simulink model "boat_control"  (R2018b)
settings: Solver=VariableStepAuto  StartTime=0.0  StopTime=150  RelTol=1e-3
libraries: simulink x5
settings Model: PacingRate=0.890000  Creator=davidm  LastModifiedBy=davidm

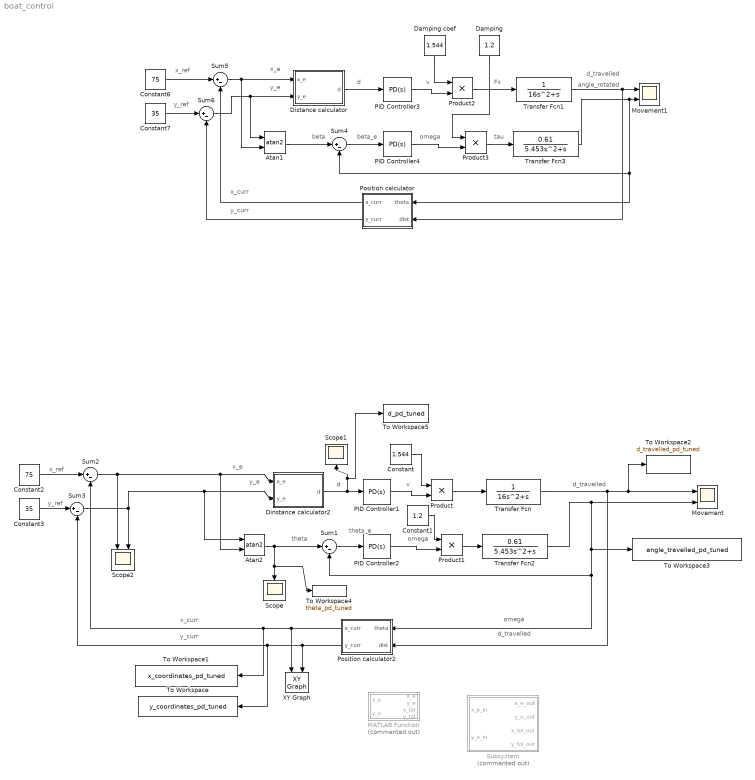
== system boat_control ==
  note: angle_rotated
  note: Fx
  note: tau
  note: y_curr
  note: x_curr
  note: omega
  note: theta
  note: d_travelled
  note: v
  note: d
  note: y_e
  note: x_e
  note: y_ref
  note: x_ref
  note: theta_e
  note: omega
  note: d_travelled
  note: y_e
  note: x_e
  note: d
  note: y_ref
  note: v
  note: d_travelled
  note: beta_e
  note: x_ref
  note: beta
  note: omega
  note: x_curr
  note: y_curr
  Atan1 : Trigonometry  Operator=atan2
  Atan2 : Trigonometry  Operator=atan2
  Constant : Constant  Value=1.544
  Constant1 : Constant  Value=1.2
  Constant2 : Constant  Value=75
  Constant3 : Constant  Value=35
  Constant6 : Constant  Value=75
  Constant7 : Constant  Value=35
  Damping : Constant  Value=1.2
  Damping coef : Constant  Value=1.544
  Dinstance calculator2 : MATLAB Function  TreatAsAtomicUnit=on
  Distance calculator : MATLAB Function  TreatAsAtomicUnit=on
  MATLAB Function : MATLAB Function  Commented=on  TreatAsAtomicUnit=on
  Movement : Scope  NumInputPorts=2
  Movement1 : Scope  NumInputPorts=2
  PID Controller1 : simulink/Continuous/PID Controller  Controller=PD  Form=Parallel  TimeDomain=Continuous-time  SampleTime=-1  IntegratorMethod=Forward Euler  FilterMethod=Forward Euler  ControllerParametersSource=internal  P=0.115276413128131  I=0.00135505762416607  D=0.95237367994795  UseFilter=on  N=1.3850682547936  TunerSelectOption=Transfer Function Based (PID Tuner App)  InitialConditionSource=internal  InitialConditionForIntegrator=0  InitialConditionForFilter=0  DifferentiatorICPrevScaledInput=0  ExternalReset=none  TrackingMode=off  Kt=1  LimitOutput=off  UpperSaturationLimit=inf  LowerSaturationLimit=-inf  LinearizeAsGain=on  AntiWindupMode=clamping  Kb=1  POutMin=[]  POutMax=[]  IOutMin=[]  IOutMax=[]  DOutMin=[]  DOutMax=[]  NOutMin=[]  NOutMax=[]  SumOutMin=[]  SumOutMax=[]  SaturationOutMin=[]  SaturationOutMax=[]  PParamMin=[]  PParamMax=[]  IParamMin=[]  IParamMax=[]  DParamMin=[]  DParamMax=[]  NParamMin=[]  NParamMax=[]  KbParamMin=[]  KbParamMax=[]  KtParamMin=[]  KtParamMax=[]  KbOutMin=[]  KbOutMax=[]  KtOutMin=[]  KtOutMax=[]  IntegratorOutMin=[]  IntegratorOutMax=[]  FilterOutMin=[]  FilterOutMax=[]  SumI1OutMin=[]  SumI1OutMax=[]  SumI2OutMin=[]  SumI2OutMax=[]  SumI3OutMin=[]  SumI3OutMax=[]  SumI4OutMin=[]  SumI4OutMax=[]  SumDOutMin=[]  SumDOutMax=[]  DifferentiatorOutMin=[]  DifferentiatorOutMax=[]  FilterDiffOutCoefMin=[]  FilterDiffOutCoefMax=[]  ReciprocalOutMin=[]  ReciprocalOutMax=[]  SumDenOutMin=[]  SumDenOutMax=[]  SumNumOutMin=[]  SumNumOutMax=[]  DivideOutMin=[]  DivideOutMax=[]  IntegratorContinuousStateAttributes=''  IntegratorStateMustResolveToSignalObject=off  IntegratorRTWStateStorageClass=Auto  FilterContinuousStateAttributes=''  FilterStateMustResolveToSignalObject=off  FilterRTWStateStorageClass=Auto  ParallelPVariant=InternalParameters  IdealPVariant=Disabled  IVariant=Disabled  DVariant=InternalParameters  IntegratorVariant=Disabled  SatVariant=Disabled  AWVariant=Disabled  PCopyVariant=Disabled  TRVariant=Disabled  FdbkBlocksVariant=Forward  IdealPFdbkVariant=Disabled  SatFdbkVariant=Disabled  DerivativeFilterVariant=ContFilter  NVariant=InternalParameters  NCopyVariant=Disabled  FilterICVariant=InternalICsFilter  IntegratorICVariant=Disabled  ExternalResetVariant=Disabled  TRSumVariant=Passthrough  SumFdbkVariant=Disabled  SumVariant=Sum_PD
  PID Controller2 : simulink/Continuous/PID Controller  Controller=PD  Form=Parallel  TimeDomain=Continuous-time  SampleTime=-1  IntegratorMethod=Forward Euler  FilterMethod=Forward Euler  ControllerParametersSource=internal  P=0.646512806885205  I=0.022298668264277  D=1.82036961249766  UseFilter=on  N=4.06401835259447  TunerSelectOption=Transfer Function Based (PID Tuner App)  InitialConditionSource=internal  InitialConditionForIntegrator=0  InitialConditionForFilter=0  DifferentiatorICPrevScaledInput=0  ExternalReset=none  TrackingMode=off  Kt=1  LimitOutput=off  UpperSaturationLimit=inf  LowerSaturationLimit=-inf  LinearizeAsGain=off  AntiWindupMode=clamping  Kb=1  POutMin=[]  POutMax=[]  IOutMin=[]  IOutMax=[]  DOutMin=[]  DOutMax=[]  NOutMin=[]  NOutMax=[]  SumOutMin=[]  SumOutMax=[]  SaturationOutMin=[]  SaturationOutMax=[]  PParamMin=[]  PParamMax=[]  IParamMin=[]  IParamMax=[]  DParamMin=[]  DParamMax=[]  NParamMin=[]  NParamMax=[]  KbParamMin=[]  KbParamMax=[]  KtParamMin=[]  KtParamMax=[]  KbOutMin=[]  KbOutMax=[]  KtOutMin=[]  KtOutMax=[]  IntegratorOutMin=[]  IntegratorOutMax=[]  FilterOutMin=[]  FilterOutMax=[]  SumI1OutMin=[]  SumI1OutMax=[]  SumI2OutMin=[]  SumI2OutMax=[]  SumI3OutMin=[]  SumI3OutMax=[]  SumI4OutMin=[]  SumI4OutMax=[]  SumDOutMin=[]  SumDOutMax=[]  DifferentiatorOutMin=[]  DifferentiatorOutMax=[]  FilterDiffOutCoefMin=[]  FilterDiffOutCoefMax=[]  ReciprocalOutMin=[]  ReciprocalOutMax=[]  SumDenOutMin=[]  SumDenOutMax=[]  SumNumOutMin=[]  SumNumOutMax=[]  DivideOutMin=[]  DivideOutMax=[]  IntegratorContinuousStateAttributes=''  IntegratorStateMustResolveToSignalObject=off  IntegratorRTWStateStorageClass=Auto  FilterContinuousStateAttributes=''  FilterStateMustResolveToSignalObject=off  FilterRTWStateStorageClass=Auto  ParallelPVariant=InternalParameters  IdealPVariant=Disabled  IVariant=Disabled  DVariant=InternalParameters  IntegratorVariant=Disabled  SatVariant=Disabled  AWVariant=Disabled  PCopyVariant=Disabled  TRVariant=Disabled  FdbkBlocksVariant=Forward  IdealPFdbkVariant=Disabled  SatFdbkVariant=Disabled  DerivativeFilterVariant=ContFilter  NVariant=InternalParameters  NCopyVariant=Disabled  FilterICVariant=InternalICsFilter  IntegratorICVariant=Disabled  ExternalResetVariant=Disabled  TRSumVariant=Passthrough  SumFdbkVariant=Disabled  SumVariant=Sum_PD
  PID Controller3 : simulink/Continuous/PID Controller  Controller=PD  Form=Parallel  TimeDomain=Continuous-time  SampleTime=-1  IntegratorMethod=Forward Euler  FilterMethod=Forward Euler  ControllerParametersSource=internal  P=0.0932700762153962  I=0.00135505762416607  D=1.11983436282053  UseFilter=on  N=0.405940642828316  TunerSelectOption=Transfer Function Based (PID Tuner App)  InitialConditionSource=internal  InitialConditionForIntegrator=0  InitialConditionForFilter=0  DifferentiatorICPrevScaledInput=0  ExternalReset=none  TrackingMode=off  Kt=1  LimitOutput=off  UpperSaturationLimit=inf  LowerSaturationLimit=-inf  LinearizeAsGain=on  AntiWindupMode=clamping  Kb=1  POutMin=[]  POutMax=[]  IOutMin=[]  IOutMax=[]  DOutMin=[]  DOutMax=[]  NOutMin=[]  NOutMax=[]  SumOutMin=[]  SumOutMax=[]  SaturationOutMin=[]  SaturationOutMax=[]  PParamMin=[]  PParamMax=[]  IParamMin=[]  IParamMax=[]  DParamMin=[]  DParamMax=[]  NParamMin=[]  NParamMax=[]  KbParamMin=[]  KbParamMax=[]  KtParamMin=[]  KtParamMax=[]  KbOutMin=[]  KbOutMax=[]  KtOutMin=[]  KtOutMax=[]  IntegratorOutMin=[]  IntegratorOutMax=[]  FilterOutMin=[]  FilterOutMax=[]  SumI1OutMin=[]  SumI1OutMax=[]  SumI2OutMin=[]  SumI2OutMax=[]  SumI3OutMin=[]  SumI3OutMax=[]  SumI4OutMin=[]  SumI4OutMax=[]  SumDOutMin=[]  SumDOutMax=[]  DifferentiatorOutMin=[]  DifferentiatorOutMax=[]  FilterDiffOutCoefMin=[]  FilterDiffOutCoefMax=[]  ReciprocalOutMin=[]  ReciprocalOutMax=[]  SumDenOutMin=[]  SumDenOutMax=[]  SumNumOutMin=[]  SumNumOutMax=[]  DivideOutMin=[]  DivideOutMax=[]  IntegratorContinuousStateAttributes=''  IntegratorStateMustResolveToSignalObject=off  IntegratorRTWStateStorageClass=Auto  FilterContinuousStateAttributes=''  FilterStateMustResolveToSignalObject=off  FilterRTWStateStorageClass=Auto  ParallelPVariant=InternalParameters  IdealPVariant=Disabled  IVariant=Disabled  DVariant=InternalParameters  IntegratorVariant=Disabled  SatVariant=Disabled  AWVariant=Disabled  PCopyVariant=Disabled  TRVariant=Disabled  FdbkBlocksVariant=Forward  IdealPFdbkVariant=Disabled  SatFdbkVariant=Disabled  DerivativeFilterVariant=ContFilter  NVariant=InternalParameters  NCopyVariant=Disabled  FilterICVariant=InternalICsFilter  IntegratorICVariant=Disabled  ExternalResetVariant=Disabled  TRSumVariant=Passthrough  SumFdbkVariant=Disabled  SumVariant=Sum_PD
  PID Controller4 : simulink/Continuous/PID Controller  Controller=PD  Form=Parallel  TimeDomain=Continuous-time  SampleTime=-1  IntegratorMethod=Forward Euler  FilterMethod=Forward Euler  ControllerParametersSource=internal  P=0.52309312144704  I=0.022298668264277  D=2.1404544119915  UseFilter=on  N=1.19109669636036  TunerSelectOption=Transfer Function Based (PID Tuner App)  InitialConditionSource=internal  InitialConditionForIntegrator=0  InitialConditionForFilter=0  DifferentiatorICPrevScaledInput=0  ExternalReset=none  TrackingMode=off  Kt=1  LimitOutput=off  UpperSaturationLimit=inf  LowerSaturationLimit=-inf  LinearizeAsGain=off  AntiWindupMode=clamping  Kb=1  POutMin=[]  POutMax=[]  IOutMin=[]  IOutMax=[]  DOutMin=[]  DOutMax=[]  NOutMin=[]  NOutMax=[]  SumOutMin=[]  SumOutMax=[]  SaturationOutMin=[]  SaturationOutMax=[]  PParamMin=[]  PParamMax=[]  IParamMin=[]  IParamMax=[]  DParamMin=[]  DParamMax=[]  NParamMin=[]  NParamMax=[]  KbParamMin=[]  KbParamMax=[]  KtParamMin=[]  KtParamMax=[]  KbOutMin=[]  KbOutMax=[]  KtOutMin=[]  KtOutMax=[]  IntegratorOutMin=[]  IntegratorOutMax=[]  FilterOutMin=[]  FilterOutMax=[]  SumI1OutMin=[]  SumI1OutMax=[]  SumI2OutMin=[]  SumI2OutMax=[]  SumI3OutMin=[]  SumI3OutMax=[]  SumI4OutMin=[]  SumI4OutMax=[]  SumDOutMin=[]  SumDOutMax=[]  DifferentiatorOutMin=[]  DifferentiatorOutMax=[]  FilterDiffOutCoefMin=[]  FilterDiffOutCoefMax=[]  ReciprocalOutMin=[]  ReciprocalOutMax=[]  SumDenOutMin=[]  SumDenOutMax=[]  SumNumOutMin=[]  SumNumOutMax=[]  DivideOutMin=[]  DivideOutMax=[]  IntegratorContinuousStateAttributes=''  IntegratorStateMustResolveToSignalObject=off  IntegratorRTWStateStorageClass=Auto  FilterContinuousStateAttributes=''  FilterStateMustResolveToSignalObject=off  FilterRTWStateStorageClass=Auto  ParallelPVariant=InternalParameters  IdealPVariant=Disabled  IVariant=Disabled  DVariant=InternalParameters  IntegratorVariant=Disabled  SatVariant=Disabled  AWVariant=Disabled  PCopyVariant=Disabled  TRVariant=Disabled  FdbkBlocksVariant=Forward  IdealPFdbkVariant=Disabled  SatFdbkVariant=Disabled  DerivativeFilterVariant=ContFilter  NVariant=InternalParameters  NCopyVariant=Disabled  FilterICVariant=InternalICsFilter  IntegratorICVariant=Disabled  ExternalResetVariant=Disabled  TRSumVariant=Passthrough  SumFdbkVariant=Disabled  SumVariant=Sum_PD
  Position calculator : MATLAB Function  TreatAsAtomicUnit=on
  Position calculator2 : MATLAB Function  TreatAsAtomicUnit=on
  Product{,1..3} (4 alike) : Product
  Scope : Scope
  Scope1 : Scope
  Scope2 : Scope  NumInputPorts=2
  Subsystem : Subsystem  Commented=on
  Sum{1..6} (6 alike) : Sum  Inputs=|+-
  To Workspace : ToWorkspace  VariableName=y_coordinates_pd_tuned  SaveFormat=Timeseries  SampleTime=-1
  To Workspace1 : ToWorkspace  VariableName=x_coordinates_pd_tuned  SaveFormat=Timeseries  SampleTime=-1
  To Workspace2 : ToWorkspace  VariableName=d_travelled_pd_tuned  SaveFormat=Timeseries  SampleTime=-1
  To Workspace3 : ToWorkspace  VariableName=angle_travelled_pd_tuned  SaveFormat=Timeseries  SampleTime=-1
  To Workspace4 : ToWorkspace  VariableName=theta_pd_tuned  SaveFormat=Timeseries  SampleTime=-1
  To Workspace5 : ToWorkspace  VariableName=d_pd_tuned  SaveFormat=Timeseries  SampleTime=-1
  Transfer Fcn : TransferFcn  Denominator=[16 1 0]
  Transfer Fcn1 : TransferFcn  Denominator=[16 1 0]
  Transfer Fcn2 : TransferFcn  Numerator=[0.61]  Denominator=[5.453 1 0]
  Transfer Fcn3 : TransferFcn  Numerator=[0.61]  Denominator=[5.453 1 0]
  XY Graph : simulink/Sinks/XY Graph  xmin=0  xmax=5000  ymin=-150  ymax=150  st=-1
  wires:
  PID Controller1/1 -> Product/2
  Constant3/1 -> Sum3/1
  Constant2/1 -> Sum2/1
  Dinstance calculator2/1(d) -> PID Controller1/1, To Workspace5/1, Scope1/1
  Position calculator2/1(x_curr) -> XY Graph/1, To Workspace1/1, Sum2/2
  Position calculator2/2(y_curr) -> XY Graph/2, To Workspace/1, Sum3/2
  Transfer Fcn2/1 -> To Workspace3/1, Sum1/2, Position calculator2/1(theta), Movement/2
  Transfer Fcn/1 -> Position calculator2/2(dist), To Workspace2/1, Movement/1
  Product/1 -> Transfer Fcn/1
  Constant/1 -> Product/1
  Product1/1 -> Transfer Fcn2/1
  PID Controller2/1 -> Product1/2
  Constant1/1 -> Product1/1
  Atan2/1 -> Scope/1, To Workspace4/1, Sum1/1
  Sum1/1 -> PID Controller2/1
  Sum2/1 -> Scope2/1, Atan2/2, Dinstance calculator2/1(x_e)
  Sum3/1 -> Atan2/1, Dinstance calculator2/2(y_e), Scope2/2
  Product2/1 -> Transfer Fcn1/1
  Damping/1 -> Product3/1
  Sum6/1 -> Atan1/1, Distance calculator/2(y_e)
  PID Controller4/1 -> Product3/2
  Position calculator/2(y_curr) -> Sum6/2
  Transfer Fcn3/1 -> Movement1/2, Sum4/2, Position calculator/1(theta)
  Transfer Fcn1/1 -> Position calculator/2(dist), Movement1/1
  Product3/1 -> Transfer Fcn3/1
  PID Controller3/1 -> Product2/2
  Constant6/1 -> Sum5/1
  Damping coef/1 -> Product2/1
  Distance calculator/1(d) -> PID Controller3/1
  Atan1/1 -> Sum4/1
  Constant7/1 -> Sum6/1
  Sum4/1 -> PID Controller4/1
  Position calculator/1(x_curr) -> Sum5/2
  Sum5/1 -> Atan1/2, Distance calculator/1(x_e)

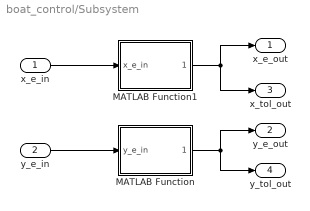
== system boat_control/Subsystem ==
  x_e_in : Inport
  y_e_in : Inport  Port=2
  MATLAB Function : MATLAB Function  TreatAsAtomicUnit=on
  MATLAB Function1 : MATLAB Function  TreatAsAtomicUnit=on
  x_e_out : Outport
  y_e_out : Outport  Port=2
  x_tol_out : Outport  Port=3
  y_tol_out : Outport  Port=4
  wires:
  x_e_in/1 -> MATLAB Function1/1(x_e_in)
  y_e_in/1 -> MATLAB Function/1(y_e_in)
  MATLAB Function/1(y_tol_out) -> y_e_out/1, y_tol_out/1
  MATLAB Function1/1(x_tol_out) -> x_tol_out/1, x_e_out/1

== matlab function boat_control/Position calculator2 ==
  data: theta input; x_curr output; dist input; y_curr output
function [x_curr, y_curr]= fcn(theta, dist)

x_curr = cos(theta) * dist;
y_curr = sin(theta) * dist;

% x_curr, y_curr;

== matlab function boat_control/Dinstance calculator2 ==
  data: x_e input; d output; y_e input
    function d = fcn(x_e, y_e)

dist = sqrt(x_e.^2 + y_e.^2)

d= dist;

== matlab function boat_control/MATLAB Function ==
  data: x_e input; x_e output; y_e input; y_e output; x_tol output; y_tol output
function [x_e, y_e, x_tol, y_tol]= fcn(x_e, y_e)

if x_e < 1 && y_e < 1
    x_tol = 0;
    y_tol = 0;
else
    x_tol = x_e;
    y_tol = y_e;
end

== matlab function boat_control/Subsystem/MATLAB Function ==
  data: y_e_in input; y_tol_out output
function y_tol_out = fcn(y_e_in)

if y_e_in <= 5
    y_tol_out = 0;
else
    y_tol_out = y_e_in;
end

== matlab function boat_control/Subsystem/MATLAB Function1 ==
  data: x_e_in input; x_tol_out output
function x_tol_out = fcn(x_e_in)

if x_e_in <= 5
    x_tol_out = 0;
else
    x_tol_out = x_e_in;
end

== matlab function boat_control/Distance calculator ==
  data: x_e input; d output; y_e input
function d = fcn(x_e, y_e)

dist = sqrt(x_e.^2 + y_e.^2)

d= dist;

== matlab function boat_control/Position calculator ==
  data: theta input; x_curr output; dist input; y_curr output
function [x_curr, y_curr]= fcn(theta, dist)

x_curr = cos(theta) * dist;
y_curr = sin(theta) * dist;

% x_curr, y_curr;
